simulink subsystem "circularBufferDPRAM"  (R2021a)
settings: Solver=VariableStepAuto  StartTime=0.0  StopTime=10.0  RelTol=1e-3
undefined symbols (not defined in the file or in its folder): modelParams
libraries: hdlsllib x1, simulink x1
settings Model: Creator=trevor  LastModifiedBy=Ross_admin

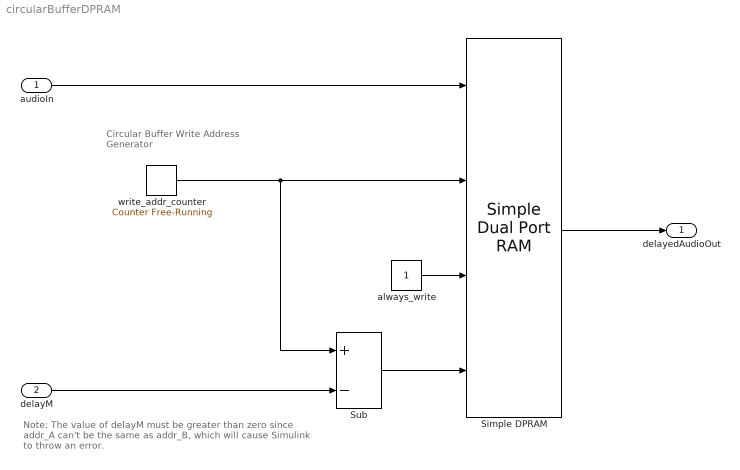
== system circularBufferDPRAM ==
  note: Note: The value of delayM must be greater than zero
      | since addr_A can't be the same as addr_B, which will cause
      | Simulink to throw an error.
  note: Circular Buffer
      | Write Address Generator
  audioIn : Inport
  delayM : Inport  Port=2  OutMin=1
  Simple DPRAM : hdlsllib/HDL RAMs/Simple Dual Port RAM  ram_size=modelParams.dpramAddressSize
      settings: SourceProductBaseCode=SL
  Sub : Sum  Inputs=+-  OutDataTypeStr=Inherit: Same as first input
  always_write : Constant  OutDataTypeStr=boolean  SampleTime=modelParams.audio.samplePeriod
  write_addr_counter : simulink/Sources/Counter Free-Running  NumBits=modelParams.dpramAddressSize  tsamp=modelParams.audio.samplePeriod
  delayedAudioOut : Outport
  wires:
  write_addr_counter/1 -> Simple DPRAM/2, Sub/1
  delayM/1 -> Sub/2
  Sub/1 -> Simple DPRAM/4
  audioIn/1 -> Simple DPRAM/1
  Simple DPRAM/1 -> delayedAudioOut/1
  always_write/1 -> Simple DPRAM/3
